simulink model "lab3sim"  (R2023b)
settings: Solver=FixedStepAuto  StartTime=0.0  StopTime=stop_time  FixedStep=0.001  RelTol=1e-3
values from neighbouring files (symbols this model uses):
  a = 2    [lab3.m]
  B = 10    [lab3.m]
  e0 = 10    [lab3.m]
  eprim0 = 0    [lab3.m]
  k1 = 2    [lab3.m]
  k2 = 1    [lab3.m]
  T = 2    [lab3.m]
  w = 0    [lab3.m]
undefined symbols (not defined in the file or in its folder): a2, a3, B2, b3, B3, e02, e03, eprim02, eprim03, k3, T3, w2
settings Model: Creator=pc  LastModifiedBy=pc

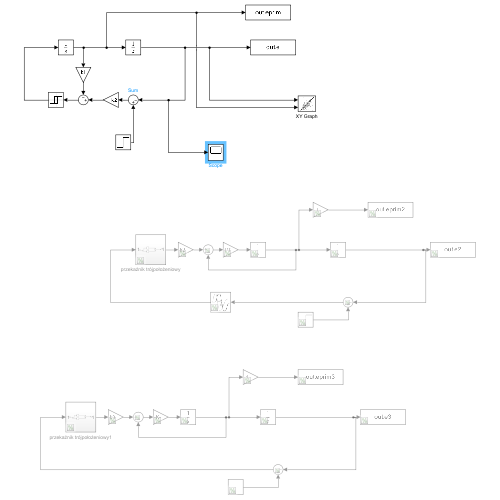
[thumbnail: Simulink's stored preview of the top-level diagram]
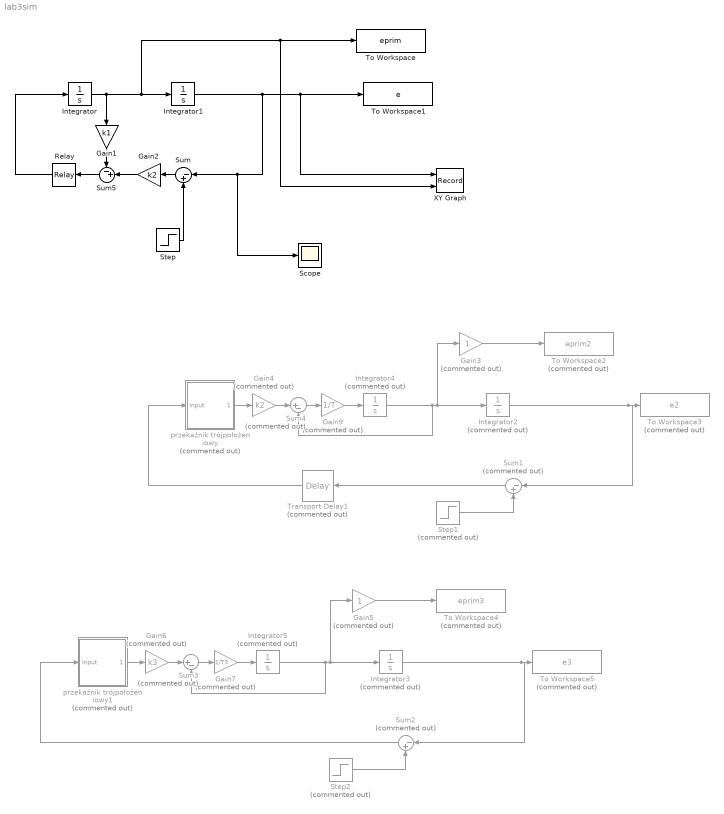
== system lab3sim ==
  Gain1 : Gain  Gain=k1
  Gain2 : Gain  Gain=k2
  Gain3 : Gain  Commented=on
  Gain4 : Gain  Commented=on  Gain=k2
  Gain5 : Gain  Commented=on
  Gain6 : Gain  Commented=on  Gain=k3
  Gain7 : Gain  Commented=on  Gain=1/T3
  Gain9 : Gain  Commented=on  Gain=1/T
  Integrator : Integrator  InitialCondition=eprim0
  Integrator1 : Integrator  InitialCondition=e0
  Integrator2 : Integrator  Commented=on  InitialCondition=e02
  Integrator3 : Integrator  Commented=on  InitialCondition=e03
  Integrator4 : Integrator  Commented=on  InitialCondition=eprim02
  Integrator5 : Integrator  Commented=on  InitialCondition=eprim03
  Relay : Relay  OnSwitchValue=a  OffSwitchValue=-a  OnOutputValue=B  OffOutputValue=-B
  Scope : Scope
  Step : Step  Time=0  After=w  SampleTime=0
  Step1 : Step  Commented=on  Time=0  After=w2  SampleTime=0
  Step2 : Step  Commented=on  Time=0  After=0  SampleTime=0
  Sum : Sum  Inputs=|-+
  Sum1 : Sum  Commented=on  Inputs=|-+
  Sum2 : Sum  Commented=on  Inputs=|-+
  Sum3 : Sum  Commented=on  Inputs=|+-
  Sum4 : Sum  Commented=on  Inputs=|+-
  Sum5 : Sum  Inputs=-+|
  To Workspace : ToWorkspace  VariableName=eprim  SaveFormat=Timeseries  SampleTime=-1
  To Workspace1 : ToWorkspace  VariableName=e  SaveFormat=Timeseries  SampleTime=-1
  To Workspace2 : ToWorkspace  Commented=on  VariableName=eprim2  SaveFormat=Timeseries  SampleTime=-1
  To Workspace3 : ToWorkspace  Commented=on  VariableName=e2  SaveFormat=Timeseries  SampleTime=-1
  To Workspace4 : ToWorkspace  Commented=on  VariableName=eprim3  SaveFormat=Timeseries  SampleTime=-1
  To Workspace5 : ToWorkspace  Commented=on  VariableName=e3  SaveFormat=Timeseries  SampleTime=-1
  Transport Delay1 : TransportDelay  Commented=on
  XY Graph : Record  FileSettingsInternal="{\"entries\":[{\"content\":{\"excelSettings\":{\"content\":{},\"type\":\"Streamout.ExcelSettings\"}},\"type\":\"Streamout.FileSettingStorage\",\"uuid\":\"\"}],\"packageUris\":[\"http:\\/\\/schema.mathworks.com\\/mf0\\/streamout_blocks\\/R2020a\"],\"version\":\"1.0\"}"  Layout=[1 1]  SignalsInternal="{\"entries\":[{\"content\":{\"signals\":[{\"content\":{\"blockPath\":[],\"dimensions\":[1],\"domain\":\"\",\"lineColor\":\"#a2142f\",\"plots\":[ 1 ],\"port\":1,\"sid\":[\"\"],\"signalID\":1,\"signalName\":\"Integrator1\"},\"type\":\"RecordBlkView.Signal\",\"uuid\":\"\"},{\"content\":{\"blockPath\":[],\"dimensions\":[1],\"domain\":\"\",\"lineColor\":\"#139fff\",\"plots\":[ 1 ],\"port\":2,\"sid\":[\"\"],\"signalID\":2,\"signalName\":\"Integrator\"},\"type\":\"RecordBlkView.Signal\",\"uuid\":\"\"}]},\"type\":\"RecordBlkView.InputSignals\",\"uuid\":\"\"}],\"packageUris\":[\"http:\\/\\/schema.mathworks.com\\/mf0\\/streamout_blocks\\/R2020a\"],\"version\":\"1.0\"}"  VisualizationBindings="{\"xyplotplugin\":{\"info\":[{\"series\":[{\"bindingParametersList\":[{\"parameter\":\"X-Axis\",\"signalID\":1,\"signalName\":\"Integrator1\"},{\"parameter\":\"Y-Axis\",\"signalID\":2,\"signalName\":\"Integrator\"}],\"seriesID\":0}],\"subplotID\":1}]}}"  CompatibilityTag=XY
  przekaźnik trójpołożeniowy : Subsystem  Commented=on
  przekaźnik trójpołożeniowy1 : Subsystem  Commented=on
  wires:
  Integrator/1 -> XY Graph/2, To Workspace/1, Integrator1/1, Gain1/1
  Integrator1/1 -> Sum/1, Scope/1, XY Graph/1, To Workspace1/1
  Relay/1 -> Integrator/1
  Sum/1 -> Gain2/1
  Step/1 -> Sum/2
  Gain3/1 -> To Workspace2/1
  Step1/1 -> Sum1/2
  Integrator4/1 -> Sum4/2, Integrator2/1, Gain3/1
  przekaźnik trójpołożeniowy/1(Output) -> Gain4/1
  Gain4/1 -> Sum4/1
  Sum4/1 -> Gain9/1
  Gain9/1 -> Integrator4/1
  Integrator2/1 -> Sum1/1, To Workspace3/1
  Sum1/1 -> Transport Delay1/1
  Transport Delay1/1 -> przekaźnik trójpołożeniowy/1(Input)
  przekaźnik trójpołożeniowy1/1(Output) -> Gain6/1
  Sum3/1 -> Gain7/1
  Gain7/1 -> Integrator5/1
  Integrator3/1 -> Sum2/1, To Workspace5/1
  Gain6/1 -> Sum3/1
  Integrator5/1 -> Sum3/2, Integrator3/1, Gain5/1
  Step2/1 -> Sum2/2
  Sum2/1 -> przekaźnik trójpołożeniowy1/1(Input)
  Gain5/1 -> To Workspace4/1
  Gain2/1 -> Sum5/2
  Sum5/1 -> Relay/1
  Gain1/1 -> Sum5/1

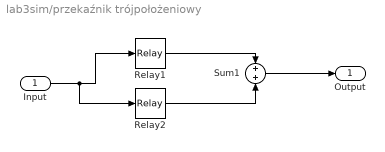
== system lab3sim/przekaźnik trójpołożeniowy ==
  Input : Inport
  Relay1 : Relay  OnSwitchValue=a2  OffSwitchValue=a2  OnOutputValue=B2
  Relay2 : Relay  OnSwitchValue=-a2  OffSwitchValue=-a2  OnOutputValue=0  OffOutputValue=-B2
  Sum1 : Sum  Inputs=+|+
  Output : Outport
  wires:
  Input/1 -> Relay2/1, Relay1/1
  Relay2/1 -> Sum1/2
  Sum1/1 -> Output/1
  Relay1/1 -> Sum1/1

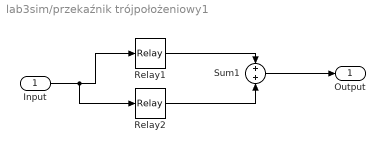
== system lab3sim/przekaźnik trójpołożeniowy1 ==
  Input : Inport
  Relay1 : Relay  OnSwitchValue=a3  OffSwitchValue=b3  OnOutputValue=B3
  Relay2 : Relay  OnSwitchValue=-b3  OffSwitchValue=-a3  OnOutputValue=0  OffOutputValue=-B3
  Sum1 : Sum  Inputs=+|+
  Output : Outport
  wires:
  Input/1 -> Relay2/1, Relay1/1
  Relay2/1 -> Sum1/2
  Sum1/1 -> Output/1
  Relay1/1 -> Sum1/1
